simulink subsystem "Dynamic_System"  (R2025b)
settings: Solver=VariableStepAuto  StartTime=0.0  StopTime=10.0  RelTol=1e-3
values from neighbouring files (symbols this model uses):
  Airbrake_CoefficientsTable = [ ... (first row only)    [data.m]
  Fin_CrossSectionArea = 0.0007    [data.m]
  Physics_Gravity = 9.81    [data.m]
  Physics_TurbulenceFactor = 0    [data.m]
  Rocket_CenterOfGravityLookupTable = [ ... (first row only)    [data.m]
  Rocket_CrossSectionArea = 0.01558    [data.m]
  Rocket_DragCoefficient = 0.461    [data.m]
  Rocket_InertiaTensorLookupTable = [ ... (first row only)    [data.m]
  Rocket_MassLookupTable = [ ... (first row only)    [data.m]
  Rocket_ThrustLookupTable = [ ... (first row only)    [data.m]
  Startup_Delay = 2.0    (= 2)    [data.m]
libraries: aerolibasang x1, simulink x1, aerolibatmos2 x1, aerolibobsolete x1, matrix_library x1
settings Model: Creator=Filip  LastModifiedBy=Filip

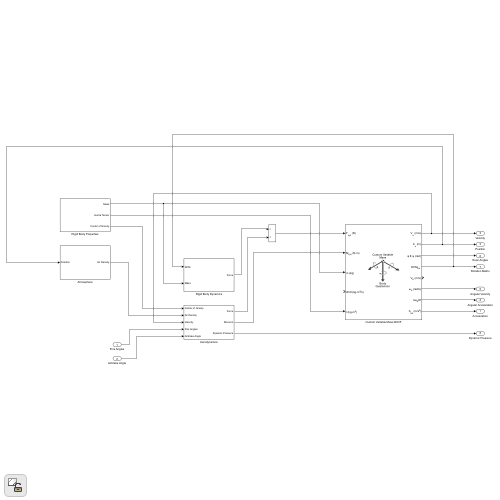
[thumbnail: Simulink's stored preview of the top-level diagram]
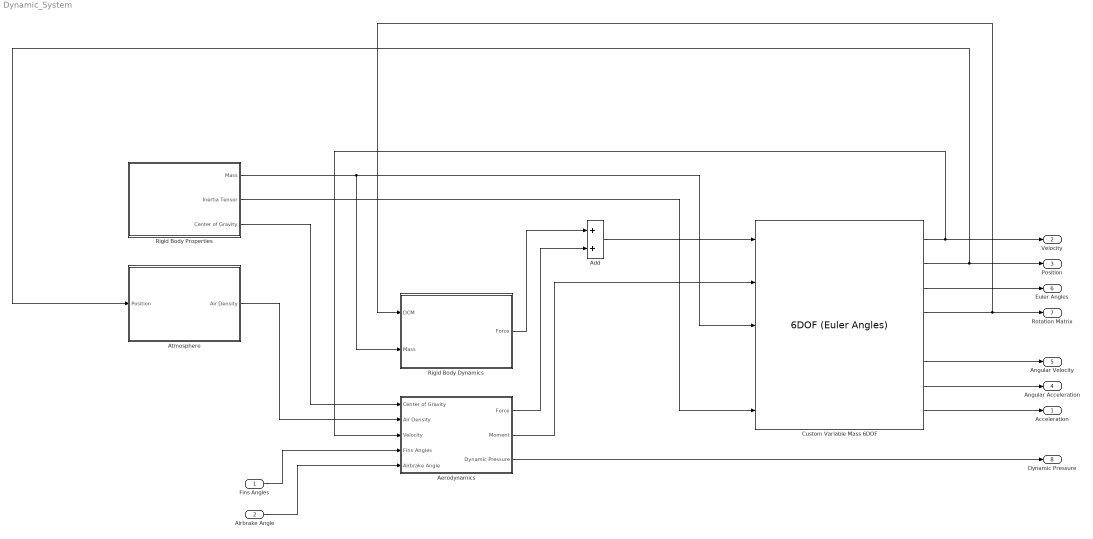
== system Dynamic_System ==
  Fins Angles : Inport
  Airbrake Angle : Inport  Port=2
  Add : Sum
  Aerodynamics : Subsystem
  Atmosphere : Subsystem
  Custom Variable Mass 6DOF : aerolibobsolete/6DOF (Euler Angles)  units=Metric (MKS)  mtype=Custom Variable  rep=Quaternion  xme_0=[0 0 0]  Vm_0=[0 0 0]  eul_0=[0 0 0]  pm_0=[0 0 0]  mass_0=1.0  mass_e=0.5  mass_f=2.0  inertia=eye(3)  inertia_e=eye(3)  inertia_f=2*eye(3)  k_quat=1.0  vre_flag=off  abi_flag=off  aMode=0  xme_statename=''  Vm_statename=''  eul_statename=''  quat_statename=''  pm_statename=''  mass_statename=''
  Rigid Body Dynamics : Subsystem
  Rigid Body Properties : Subsystem
  Acceleration : Outport
  Velocity : Outport  Port=2
  Position : Outport  Port=3
  Angular Acceleration : Outport  Port=4
  Angular Velocity : Outport  Port=5
  Euler Angles : Outport  Port=6
  Rotation Matrix : Outport  Port=7
  Dynamic Pressure : Outport  Port=8
  wires:
  Custom Variable Mass 6DOF/2 -> Atmosphere/1(Position), Position/1
  Custom Variable Mass 6DOF/3 -> Euler Angles/1
  Custom Variable Mass 6DOF/6 -> Angular Velocity/1
  Custom Variable Mass 6DOF/8 -> Acceleration/1
  Rigid Body Properties/2(Inertia Tensor) -> Custom Variable Mass 6DOF/5
  Custom Variable Mass 6DOF/4 -> Rigid Body Dynamics/1(DCM), Rotation Matrix/1
  Aerodynamics/1(Force) -> Add/2
  Aerodynamics/2(Moment) -> Custom Variable Mass 6DOF/2
  Fins Angles/1 -> Aerodynamics/4(Fins Angles)
  Custom Variable Mass 6DOF/7 -> Angular Acceleration/1
  Rigid Body Dynamics/1(Force) -> Add/1
  Add/1 -> Custom Variable Mass 6DOF/1
  Airbrake Angle/1 -> Aerodynamics/5(Airbrake Angle)
  Rigid Body Properties/1(Mass) -> Rigid Body Dynamics/2(Mass), Custom Variable Mass 6DOF/3
  Custom Variable Mass 6DOF/1 -> Aerodynamics/3(Velocity), Velocity/1
  Atmosphere/1(Air Density) -> Aerodynamics/2(Air Density)
  Rigid Body Properties/3(Center of Gravity) -> Aerodynamics/1(Center of Gravity)
  Aerodynamics/3(Dynamic Pressure) -> Dynamic Pressure/1

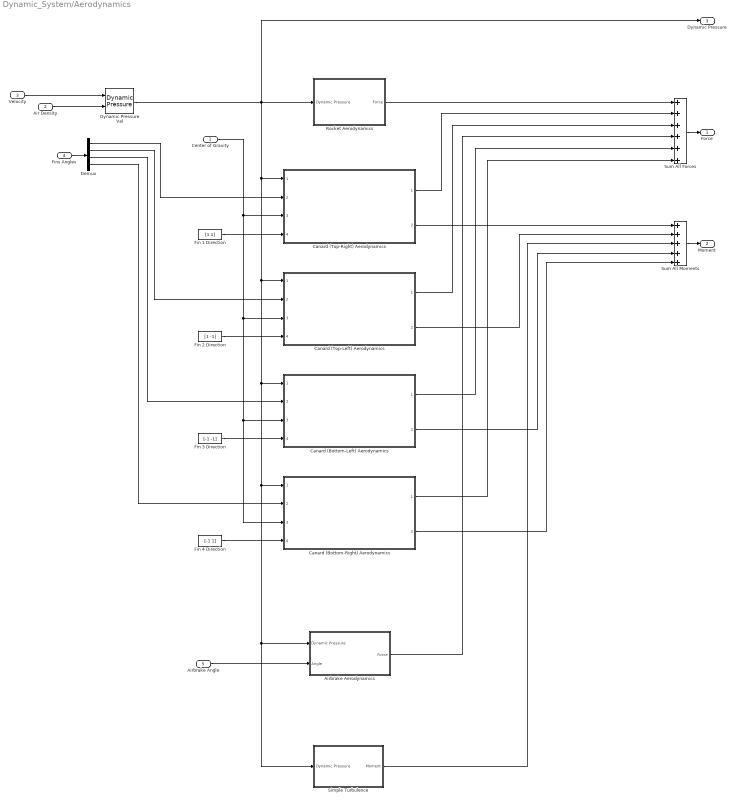
== system Dynamic_System/Aerodynamics ==
  Center of Gravity : Inport
  Air Density : Inport  Port=2
  Velocity : Inport  Port=3
  Fins Angles : Inport  Port=4
  Airbrake Angle : Inport  Port=5
  Airbrake Aerodynamics : Subsystem
  Canard (Bottom-Left) Aerodynamics : Subsystem  ReferencedSubsystem=Canard_Aerodynamics
  Canard (Bottom-Right) Aerodynamics : Subsystem  ReferencedSubsystem=Canard_Aerodynamics
  Canard (Top-Left) Aerodynamics : Subsystem  ReferencedSubsystem=Canard_Aerodynamics
  Canard (Top-Right) Aerodynamics : Subsystem  ReferencedSubsystem=Canard_Aerodynamics
  Demux : Demux
  Dynamic Pressure Val : aerolibasang/Dynamic Pressure
  Fin 1 Direction : Constant  Value=[1 1]
  Fin 2 Direction : Constant  Value=[1 -1]
  Fin 3 Direction : Constant  Value=[-1 -1]
  Fin 4 Direction : Constant  Value=[-1 1]
  Rocket Aerodynamics : Subsystem
  Simple Turbulence : Subsystem
  Sum All Forces : Sum  Inputs=++++++
  Sum All Moments : Sum  Inputs=+++++
  Force : Outport
  Moment : Outport  Port=2
  Dynamic Pressure : Outport  Port=3
  wires:
  Airbrake Aerodynamics/1(Force) -> Sum All Forces/4
  Airbrake Angle/1 -> Airbrake Aerodynamics/2(Angle)
  Simple Turbulence/1(Moment) -> Sum All Moments/3
  Center of Gravity/1 -> Canard (Top-Right) Aerodynamics/3, Canard (Top-Left) Aerodynamics/3, Canard (Bottom-Left) Aerodynamics/3, Canard (Bottom-Right) Aerodynamics/3
  Canard (Top-Left) Aerodynamics/2 -> Sum All Moments/2
  Canard (Top-Right) Aerodynamics/2 -> Sum All Moments/1
  Canard (Top-Left) Aerodynamics/1 -> Sum All Forces/3
  Canard (Top-Right) Aerodynamics/1 -> Sum All Forces/2
  Demux/1 -> Canard (Top-Right) Aerodynamics/2
  Demux/2 -> Canard (Top-Left) Aerodynamics/2
  Fin 2 Direction/1 -> Canard (Top-Left) Aerodynamics/4
  Fin 1 Direction/1 -> Canard (Top-Right) Aerodynamics/4
  Air Density/1 -> Dynamic Pressure Val/2
  Velocity/1 -> Dynamic Pressure Val/1
  Dynamic Pressure Val/1 -> Canard (Top-Right) Aerodynamics/1, Canard (Top-Left) Aerodynamics/1, Airbrake Aerodynamics/1(Dynamic Pressure), Simple Turbulence/1(Dynamic Pressure), Canard (Bottom-Right) Aerodynamics/1, Canard (Bottom-Left) Aerodynamics/1, Rocket Aerodynamics/1(Dynamic Pressure), Dynamic Pressure/1
  Rocket Aerodynamics/1(Force) -> Sum All Forces/1
  Fins Angles/1 -> Demux/1
  Sum All Moments/1 -> Moment/1
  Sum All Forces/1 -> Force/1
  Demux/3 -> Canard (Bottom-Left) Aerodynamics/2
  Demux/4 -> Canard (Bottom-Right) Aerodynamics/2
  Fin 3 Direction/1 -> Canard (Bottom-Left) Aerodynamics/4
  Fin 4 Direction/1 -> Canard (Bottom-Right) Aerodynamics/4
  Canard (Bottom-Left) Aerodynamics/1 -> Sum All Forces/5
  Canard (Bottom-Right) Aerodynamics/1 -> Sum All Forces/6
  Canard (Bottom-Left) Aerodynamics/2 -> Sum All Moments/4
  Canard (Bottom-Right) Aerodynamics/2 -> Sum All Moments/5

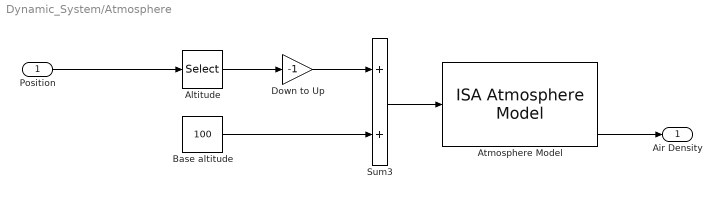
== system Dynamic_System/Atmosphere ==
  Position : Inport
  Altitude : Selector  IndexMode=Zero-based  InputPortWidth=3  IndexOptions=Index vector (dialog)  Indices=2  OutputSizes=1
  Atmosphere Model : aerolibatmos2/ISA Atmosphere Model  useExtended=off  action=Warning  custom=off  viscosityOut=off  g=9.80665  gamma=1.4  R=287.0531  L=0.0065  h_trop=11000  h_strat=20000  rho0=1.225  P0=101325  T0=288.15  h0=0  S=110.4  Tref=273.15  muref=1.716e-5
  Base altitude : Constant  Value=100
  Down to Up : Gain  Gain=-1
  Sum3 : Sum
  Air Density : Outport
  wires:
  Down to Up/1 -> Sum3/1
  Altitude/1 -> Down to Up/1
  Position/1 -> Altitude/1
  Sum3/1 -> Atmosphere Model/1
  Base altitude/1 -> Sum3/2
  Atmosphere Model/4 -> Air Density/1

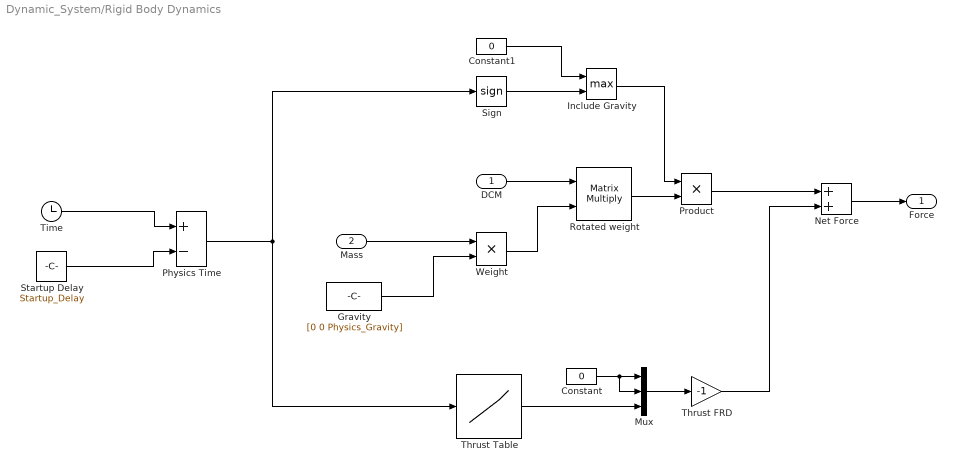
== system Dynamic_System/Rigid Body Dynamics ==
  DCM : Inport
  Mass : Inport  Port=2
  Constant : Constant  Value=0
  Constant1 : Constant  Value=0
  Gravity : Constant  Value=[0 0 Physics_Gravity]
  Include Gravity : MinMax  Function=max  Inputs=2
  Mux : Mux  Inputs=3
  Net Force : Sum
  Physics Time : Sum  Inputs=+-
  Product : Product
  Rotated weight : Product  Multiplication=Matrix(*)
  Sign : Signum
  Startup Delay : Constant  Value=Startup_Delay
  Thrust FRD : Gain  Gain=-1
  Thrust Table : Lookup_n-D  NumberOfTableDimensions=1  BreakpointsForDimension1=Rocket_ThrustLookupTable(:, 1)  Table=Rocket_ThrustLookupTable(:, 2)  ExtrapMethod=Clip  InternalRulePriority=Speed  RndMeth=Simplest
  Time : Clock
  Weight : Product
  Force : Outport
  wires:
  Thrust FRD/1 -> Net Force/2
  Mux/1 -> Thrust FRD/1
  Mass/1 -> Weight/1
  Weight/1 -> Rotated weight/2
  Constant/1 -> Mux/1, Mux/2
  Thrust Table/1 -> Mux/3
  Net Force/1 -> Force/1
  DCM/1 -> Rotated weight/1
  Gravity/1 -> Weight/2
  Time/1 -> Physics Time/1
  Startup Delay/1 -> Physics Time/2
  Physics Time/1 -> Thrust Table/1, Sign/1
  Rotated weight/1 -> Product/2
  Product/1 -> Net Force/1
  Sign/1 -> Include Gravity/2
  Include Gravity/1 -> Product/1
  Constant1/1 -> Include Gravity/1

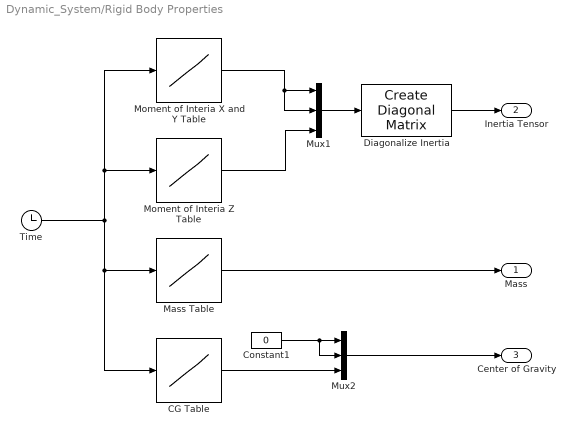
== system Dynamic_System/Rigid Body Properties ==
  CG Table : Lookup_n-D  NumberOfTableDimensions=1  BreakpointsForDimension1=Rocket_CenterOfGravityLookupTable(:, 1)  Table=Rocket_CenterOfGravityLookupTable(:, 2)  ExtrapMethod=Clip  InternalRulePriority=Speed  RndMeth=Simplest
  Constant1 : Constant  Value=0
  Diagonalize Inertia : matrix_library/Create Diagonal Matrix
  Mass Table : Lookup_n-D  NumberOfTableDimensions=1  BreakpointsForDimension1=Rocket_MassLookupTable(:, 1)  Table=Rocket_MassLookupTable(:, 2)  ExtrapMethod=Clip  InternalRulePriority=Speed  RndMeth=Simplest
  Moment of Interia X and Y Table : Lookup_n-D  NumberOfTableDimensions=1  BreakpointsForDimension1=Rocket_InertiaTensorLookupTable(:, 1)  Table=Rocket_InertiaTensorLookupTable(:, 2)  ExtrapMethod=Clip  InternalRulePriority=Speed  RndMeth=Simplest
  Moment of Interia Z Table : Lookup_n-D  NumberOfTableDimensions=1  BreakpointsForDimension1=Rocket_InertiaTensorLookupTable(:, 1)  Table=Rocket_InertiaTensorLookupTable(:, 3)  ExtrapMethod=Clip  InternalRulePriority=Speed  RndMeth=Simplest
  Mux1 : Mux  Inputs=3
  Mux2 : Mux  Inputs=3
  Time : Clock
  Mass : Outport
  Inertia Tensor : Outport  Port=2
  Center of Gravity : Outport  Port=3
  wires:
  Mux2/1 -> Center of Gravity/1
  Mux1/1 -> Diagonalize Inertia/1
  CG Table/1 -> Mux2/3
  Constant1/1 -> Mux2/1, Mux2/2
  Diagonalize Inertia/1 -> Inertia Tensor/1
  Time/1 -> Moment of Interia Z Table/1, Moment of Interia X and Y Table/1, CG Table/1, Mass Table/1
  Moment of Interia Z Table/1 -> Mux1/3
  Moment of Interia X and Y Table/1 -> Mux1/1, Mux1/2
  Mass Table/1 -> Mass/1

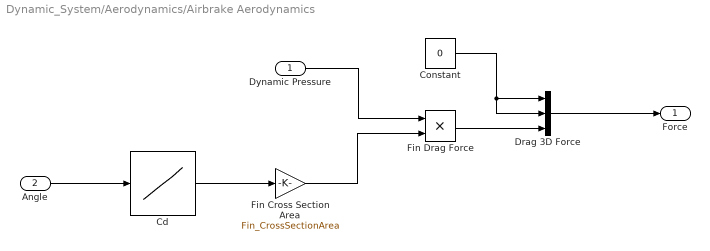
== system Dynamic_System/Aerodynamics/Airbrake Aerodynamics ==
  Dynamic Pressure : Inport
  Angle : Inport  Port=2
  Cd : Lookup_n-D  NumberOfTableDimensions=1  BreakpointsForDimension1=Airbrake_CoefficientsTable(:, 1)  Table=Airbrake_CoefficientsTable(:, 2)  ExtrapMethod=Clip  UseLastTableValue=on  InternalRulePriority=Speed  RndMeth=Simplest
  Constant : Constant  Value=0
  Drag 3D Force : Mux  Inputs=3
  Fin Cross Section Area : Gain  Gain=Fin_CrossSectionArea
  Fin Drag Force : Product
  Force : Outport
  wires:
  Constant/1 -> Drag 3D Force/1, Drag 3D Force/2
  Fin Cross Section Area/1 -> Fin Drag Force/2
  Angle/1 -> Cd/1
  Drag 3D Force/1 -> Force/1
  Dynamic Pressure/1 -> Fin Drag Force/1
  Cd/1 -> Fin Cross Section Area/1
  Fin Drag Force/1 -> Drag 3D Force/3

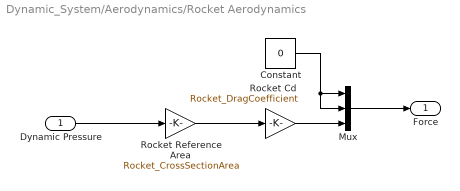
== system Dynamic_System/Aerodynamics/Rocket Aerodynamics ==
  Dynamic Pressure : Inport
  Constant : Constant  Value=0
  Mux : Mux  Inputs=3
  Rocket Cd : Gain  Gain=Rocket_DragCoefficient
  Rocket Reference Area : Gain  Gain=Rocket_CrossSectionArea
  Force : Outport
  wires:
  Mux/1 -> Force/1
  Rocket Cd/1 -> Mux/3
  Constant/1 -> Mux/2, Mux/1
  Rocket Reference Area/1 -> Rocket Cd/1
  Dynamic Pressure/1 -> Rocket Reference Area/1

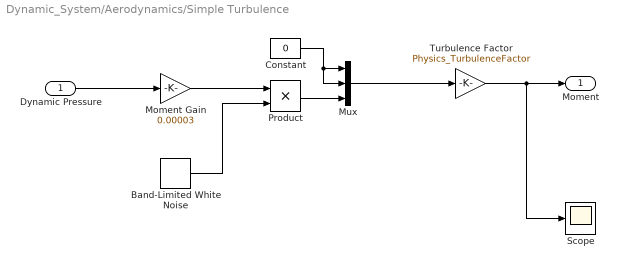
== system Dynamic_System/Aerodynamics/Simple Turbulence ==
  Dynamic Pressure : Inport
  Band-Limited White Noise : simulink/Sources/Band-Limited White Noise  Cov=[0.1]  Ts=0.1  seed=[42453]
  Constant : Constant  Value=0
  Moment Gain : Gain  Gain=0.00003
  Mux : Mux  Inputs=3
  Product : Product
  Scope : Scope
      settings: ActiveDisplayYMinimum=-1  ActiveDisplayYMaximum=1  DataLoggingVariableName=ScopeData3
  Turbulence Factor : Gain  Gain=Physics_TurbulenceFactor
  Moment : Outport
  wires:
  Turbulence Factor/1 -> Moment/1, Scope/1
  Band-Limited White Noise/1 -> Product/2
  Mux/1 -> Turbulence Factor/1
  Constant/1 -> Mux/1, Mux/2
  Product/1 -> Mux/3
  Moment Gain/1 -> Product/1
  Dynamic Pressure/1 -> Moment Gain/1
